simulink model "ekviv_prenos_nelin_2_relays_hyster"  (R2018a)
settings: Solver=VariableStepAuto  StartTime=0.0  StopTime=10.0  RelTol=1e-3
settings Model: Creator=vejvarm  LastModifiedBy=vejvarm

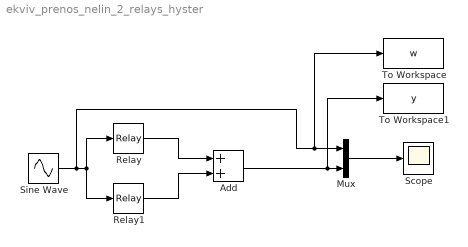
== system ekviv_prenos_nelin_2_relays_hyster ==
  Add : Sum
  Mux : Mux  Inputs=2
  Relay : Relay  OnSwitchValue=0.5  OffSwitchValue=0.5
  Relay1 : Relay  OnSwitchValue=-0.5  OffSwitchValue=-0.5  OnOutputValue=0  OffOutputValue=-1
  Scope : Scope
  Sine Wave : Sin  Amplitude=2  Frequency=2  SampleTime=0
  To Workspace : ToWorkspace  VariableName=w  SaveFormat=Timeseries  SampleTime=-1
  To Workspace1 : ToWorkspace  VariableName=y  SaveFormat=Timeseries  SampleTime=-1
  wires:
  Relay/1 -> Add/1
  Relay1/1 -> Add/2
  Sine Wave/1 -> To Workspace/1, Mux/1, Relay1/1, Relay/1
  Add/1 -> To Workspace1/1, Mux/2
  Mux/1 -> Scope/1
